simulink model "P6"  (R2023b)
settings: Solver=ode45  StartTime=0.0  StopTime=0.01  MaxStep=0.001  RelTol=1e-3
values from neighbouring files (symbols this model uses):
  C = 10e-6    (= 1e-05)    [Conv_CD_DC.m]    (also in ParametrosP6.m)
  L = 2e-3    (= 0.002)    [Conv_CD_DC.m]    (also in ParametrosP6.m)
  R = 10    [Conv_CD_DC.m]    (also in ParametrosP6.m)
  Uin = 32    [Conv_CD_DC.m]    (also in ParametrosP6.m)
settings Model: Creator=aquet  LastModifiedBy=aquet

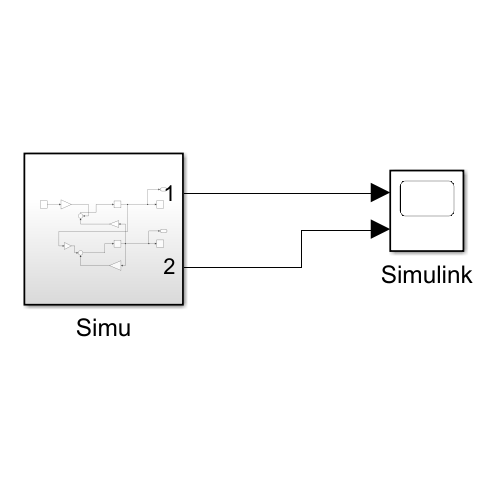
[thumbnail: Simulink's stored preview of the top-level diagram]
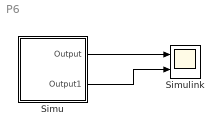
== system P6 ==
  Simu : Subsystem
  Simulink : Scope  NumInputPorts=2
  wires:
  Simu/1(Output) -> Simulink/1
  Simu/2(Output1) -> Simulink/2

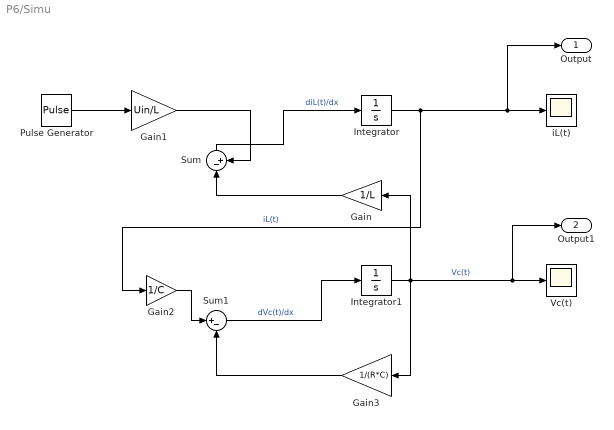
== system P6/Simu ==
  Gain : Gain  Gain=1/L
  Gain1 : Gain  Gain=Uin/L
  Gain2 : Gain  Gain=1/C
  Gain3 : Gain  Gain=1/(R*C)
  Integrator : Integrator
  Integrator1 : Integrator
  Pulse Generator : DiscretePulseGenerator  PulseType=Time based  Amplitude=0.955  Period=1e-5  PulseWidth=40
  Sum : Sum  Inputs=|-+
  Sum1 : Sum  Inputs=|+-
  Vc(t) : Scope
  iL(t) : Scope
  Output : Outport
  Output1 : Outport  Port=2
  wires:
  Pulse Generator/1 -> Gain1/1
  Sum1/1 -> Integrator1/1  "dVc(t)/dx"
  Sum/1 -> Integrator/1  "diL(t)/dx"
  Integrator1/1 -> Gain3/1, Gain/1, Output1/1, Vc(t)/1  "Vc(t)"
  Gain2/1 -> Sum1/1
  Integrator/1 -> Gain2/1, Output/1, iL(t)/1  "iL(t)"
  Gain/1 -> Sum/1
  Gain1/1 -> Sum/2
  Gain3/1 -> Sum1/2
